simulink model "practic7_4_5"  (R2020b)
settings: Solver=ode4  StartTime=0.0  StopTime=10.0  FixedStep=0.001  RelTol=1e-3
libraries: simulink x1
settings Model: Creator=yuto  LastModifiedBy=yuto
settings DataIOCC: ReturnWorkspaceOutputs=off

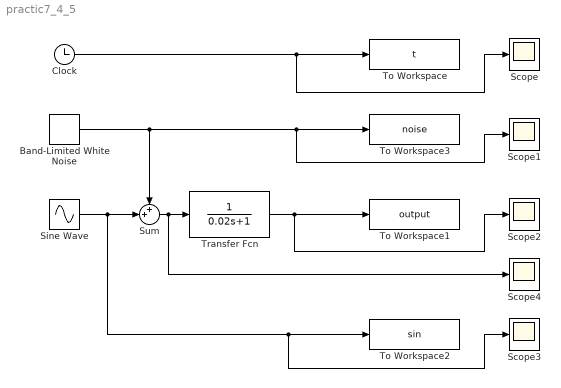
== system practic7_4_5 ==
  Band-Limited White Noise : simulink/Sources/Band-Limited White Noise  Cov=[1e-5]  Ts=0.001  seed=[23341]
  Clock : Clock
  Scope{,1..4} (5 alike) : Scope
  Sine Wave : Sin  SampleTime=0
  Sum : Sum  Inputs=++|
  To Workspace : ToWorkspace  VariableName=t  SampleTime=-1
  To Workspace1 : ToWorkspace  VariableName=output  SampleTime=-1
  To Workspace2 : ToWorkspace  VariableName=sin  SampleTime=-1
  To Workspace3 : ToWorkspace  VariableName=noise  SampleTime=-1
  Transfer Fcn : TransferFcn  Denominator=[0.02 1]
  wires:
  Band-Limited White Noise/1 -> Sum/1, Scope1/1, To Workspace3/1
  Sine Wave/1 -> Scope3/1, To Workspace2/1, Sum/2
  Sum/1 -> Scope4/1, Transfer Fcn/1
  Clock/1 -> Scope/1, To Workspace/1
  Transfer Fcn/1 -> Scope2/1, To Workspace1/1
